simulink library "INT_FlWtDet_DD"  (R2016b)
settings: Solver=VariableStepAuto  StartTime=0.0  StopTime=10.0  RelTol=1e-3
settings Model: Creator=Wei Liang  LastModifiedBy=Wei Liang

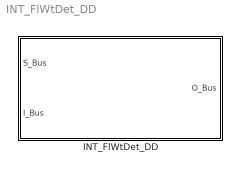
== system INT_FlWtDet_DD ==
  INT_FlWtDet_DD : Subsystem

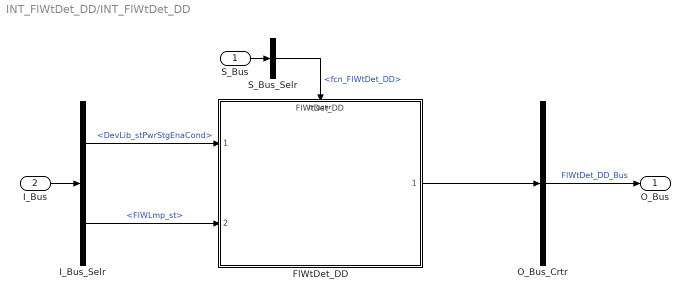
== system INT_FlWtDet_DD/INT_FlWtDet_DD ==
  S_Bus : Inport
  I_Bus : Inport  Port=2
  FlWtDet_DD : ModelReference  ModelNameDialog=FlWtDet_DD  SimulationMode=Normal  ModelReferenceVersion=1.6  TriggerPortName=function  TriggerPortTriggerType=function-call  TriggerPortStatesWhenEnabling=held
  I_Bus_Selr : BusSelector  OutputSignals=DevLib_stPwrStgEnaCond,FlWLmp_st
  O_Bus_Crtr : BusCreator  Inputs=1
  S_Bus_Selr : BusSelector  OutputSignals=fcn_FlWtDet_DD
  O_Bus : Outport
  wires:
  S_Bus_Selr/1 -> FlWtDet_DD/Trigger  "<fcn_FlWtDet_DD>"
  S_Bus/1 -> S_Bus_Selr/1
  I_Bus/1 -> I_Bus_Selr/1
  I_Bus_Selr/1 -> FlWtDet_DD/1  "<DevLib_stPwrStgEnaCond>"
  I_Bus_Selr/2 -> FlWtDet_DD/2  "<FlWLmp_st>"
  O_Bus_Crtr/1 -> O_Bus/1  "FlWtDet_DD_Bus"
  FlWtDet_DD/1 -> O_Bus_Crtr/1
